simulink model "Linearized_state_feedback"  (R2021b)
settings: Solver=VariableStepAuto  StartTime=0.0  StopTime=10  RelTol=1e-3
values from neighbouring files (symbols this model uses):
  eq = [0, 0, pi, 0]    [Linearization_comparison.m]    (also in Synthesis.m = [0, 0, -perturbation, 0]; init.m)
  K = acker(A, B, P)    [Synthesis.m]
  theta = pi    (= 3.14159265359)    [Synthesis.m]
undefined symbols (not defined in the file or in its folder): A, B
settings Model: Creator=brizio  LastModifiedBy=brizio

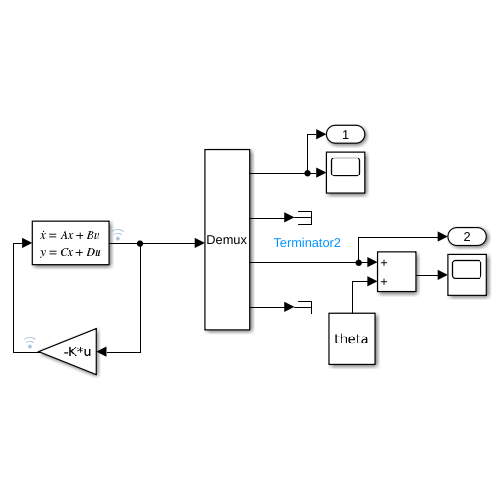
[thumbnail: Simulink's stored preview of the top-level diagram]
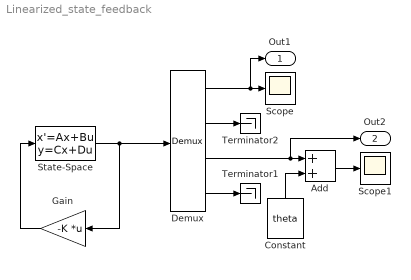
== system Linearized_state_feedback ==
  Add : Sum
  Constant : Constant  Value=theta
  Demux : Demux
      settings: DisplayOption=none
  Gain : Gain  Gain=-K  Multiplication=Matrix(K*u)
  Scope : Scope
  Scope1 : Scope
  State-Space : StateSpace  A=A  B=B  C=eye(4)  D=zeros(4, 1)  InitialCondition=eq
  Terminator1 : Terminator
  Terminator2 : Terminator
  Out1 : Outport
  Out2 : Outport  Port=2
  wires:
  State-Space/1 -> Gain/1, Demux/1
  Gain/1 -> State-Space/1
  Demux/1 -> Out1/1, Scope/1
  Demux/3 -> Out2/1, Add/1
  Demux/4 -> Terminator1/1
  Add/1 -> Scope1/1
  Constant/1 -> Add/2
  Demux/2 -> Terminator2/1
